simulink model "mdl01_IdealCtrl"  (R2022a)
settings: Solver=FixedStepAuto  StartTime=0.0  StopTime=T1  FixedStep=Ts  RelTol=1e-3
undefined symbols (not defined in the file): a, du, G1, G2, Ts, v0, x0, xt
settings Model: Creator=xiaocy  LastModifiedBy=xiaocy
settings DataIOCC: SaveOutput=off  SignalLogging=off  DSMLogging=off  SaveTime=off  ReturnWorkspaceOutputs=off

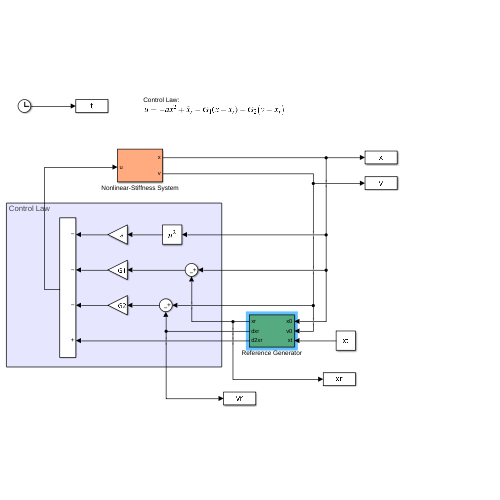
[thumbnail: Simulink's stored preview of the top-level diagram]
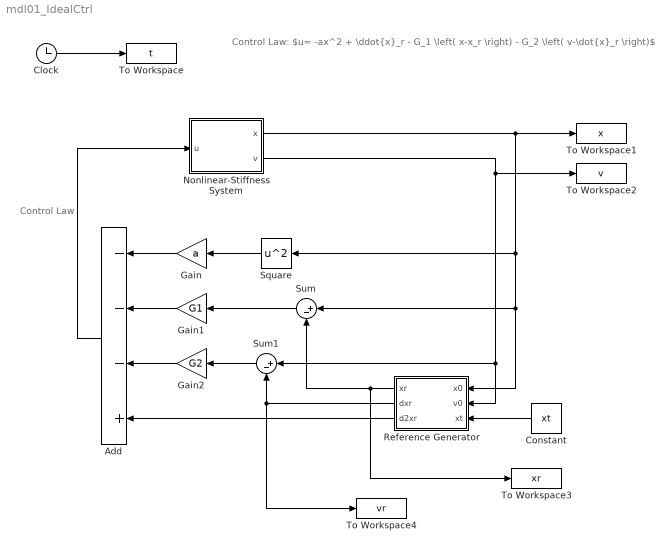
== system mdl01_IdealCtrl ==
  note: Control Law
  note: Control Law:
      | $u= -ax^2 + \ddot{x}_r - G_1 \left( x-x_r \right) - G_2 \left( v-\dot{x}_r \right)$
  Add : Sum  Inputs=---+
  Clock : Clock
  Constant : Constant  Value=xt
  Gain : Gain  Gain=a
  Gain1 : Gain  Gain=G1
  Gain2 : Gain  Gain=G2
  Nonlinear-Stiffness System : Subsystem
  Reference Generator : Subsystem
  Square : Math  Operator=square
  Sum : Sum  Inputs=|+-
  Sum1 : Sum  Inputs=|+-
  To Workspace : ToWorkspace  VariableName=t  SampleTime=Ts
  To Workspace1 : ToWorkspace  VariableName=x  SampleTime=Ts
  To Workspace2 : ToWorkspace  VariableName=v  SampleTime=Ts
  To Workspace3 : ToWorkspace  VariableName=xr  SampleTime=Ts
  To Workspace4 : ToWorkspace  VariableName=vr  SampleTime=Ts
  wires:
  Clock/1 -> To Workspace/1
  Nonlinear-Stiffness System/1(x) -> Sum/1, Reference Generator/1(x0), Square/1, To Workspace1/1
  Nonlinear-Stiffness System/2(v) -> To Workspace2/1, Sum1/1, Reference Generator/2(v0)
  Reference Generator/1(xr) -> To Workspace3/1, Sum/2
  Sum/1 -> Gain1/1
  Sum1/1 -> Gain2/1
  Reference Generator/2(dxr) -> To Workspace4/1, Sum1/2
  Square/1 -> Gain/1
  Gain/1 -> Add/1
  Gain1/1 -> Add/2
  Gain2/1 -> Add/3
  Reference Generator/3(d2xr) -> Add/4
  Add/1 -> Nonlinear-Stiffness System/1(u)
  Constant/1 -> Reference Generator/3(xt)

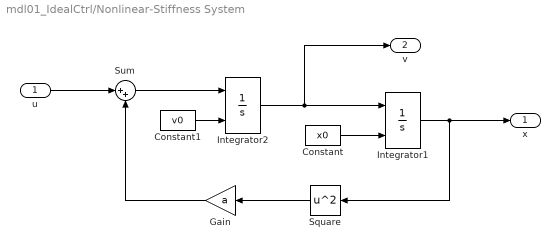
== system mdl01_IdealCtrl/Nonlinear-Stiffness System ==
  u : Inport
  Constant : Constant  Value=x0
  Constant1 : Constant  Value=v0
  Gain : Gain  Gain=a
  Integrator1 : Integrator  InitialConditionSource=external
  Integrator2 : Integrator  InitialConditionSource=external
  Square : Math  Operator=square
  Sum : Sum  Inputs=|++
  x : Outport
  v : Outport  Port=2
  wires:
  Gain/1 -> Sum/2
  Square/1 -> Gain/1
  Sum/1 -> Integrator2/1
  Integrator2/1 -> v/1, Integrator1/1
  u/1 -> Sum/1
  Integrator1/1 -> Square/1, x/1
  Constant/1 -> Integrator1/2
  Constant1/1 -> Integrator2/2

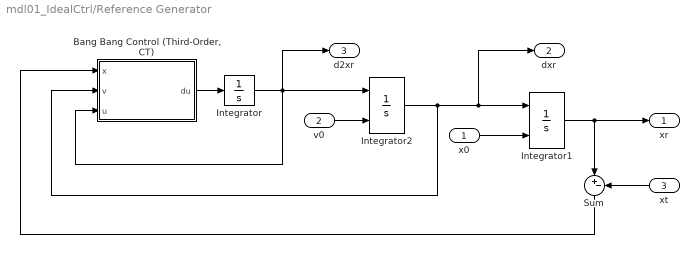
== system mdl01_IdealCtrl/Reference Generator ==
  x0 : Inport
  v0 : Inport  Port=2
  xt : Inport  Port=3
  "Bang Bang Control (Third-Order, CT)" : Subsystem  mask(Bang Bang Control){r=du}
      mask prompts: r "Actuation slope"
      mask help: Calculate command for the third-order system (series of intergrators).
      mask Display: disp('Bang-Bang\n\n(3rd, CT)')
  Integrator : Integrator
  Integrator1 : Integrator  InitialConditionSource=external
  Integrator2 : Integrator  InitialConditionSource=external
  Sum : Sum  Inputs=|+-
  xr : Outport
  dxr : Outport  Port=2
  d2xr : Outport  Port=3
  wires:
  v0/1 -> Integrator2/2
  x0/1 -> Integrator1/2
  Integrator1/1 -> xr/1, Sum/1
  Integrator2/1 -> "Bang Bang Control (Third-Order, CT)"/2(v), Integrator1/1, dxr/1
  Integrator/1 -> Integrator2/1, d2xr/1, "Bang Bang Control (Third-Order, CT)"/3(u)
  "Bang Bang Control (Third-Order, CT)"/1(du) -> Integrator/1
  xt/1 -> Sum/2
  Sum/1 -> "Bang Bang Control (Third-Order, CT)"/1(x)

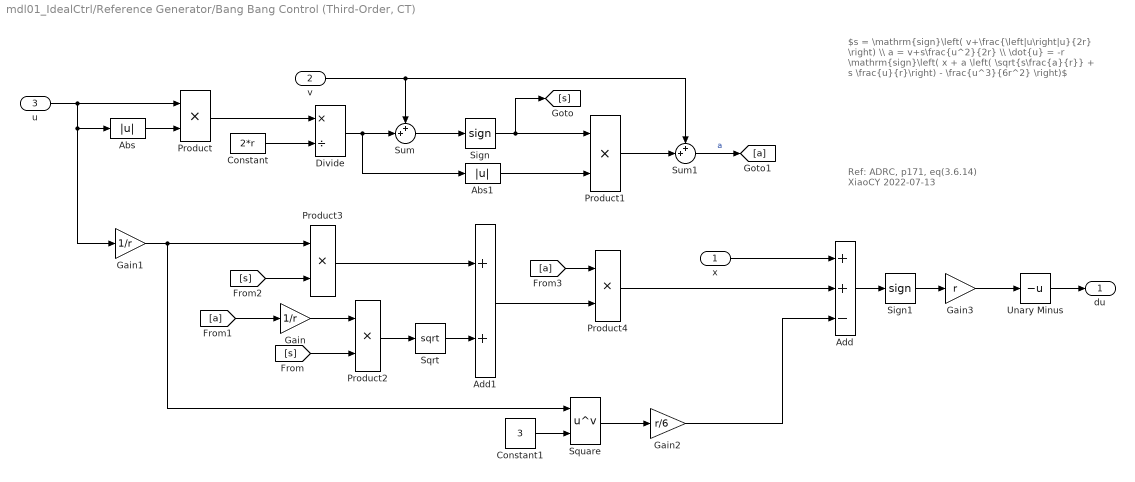
== system mdl01_IdealCtrl/Reference Generator/Bang Bang Control (Third-Order, CT) ==
  note: Ref: ADRC, p171, eq(3.6.14)
      | XiaoCY 2022-07-13
  note: $s = \mathrm{sign}\left( v+\frac{\left|u\right|u}{2r} \right) \\ a = v+s\frac{u^2}{2r} \\ \dot{u} = -r \mathrm{sign}\left( x + a \left( \sqrt{s\frac{a}{r}} + s \frac{u}{r}\right) - \frac{u^3}{6r^2} \right)$
  x : Inport
  v : Inport  Port=2
  u : Inport  Port=3
  Abs : Abs  SaturateOnIntegerOverflow=off
  Abs1 : Abs  SaturateOnIntegerOverflow=off
  Add : Sum  Inputs=++-
  Add1 : Sum
  Constant : Constant  Value=2*r
  Constant1 : Constant  Value=3
  Divide : Product  Inputs=*/
  Gain : Gain  Gain=1/r
  Gain1 : Gain  Gain=1/r
  Gain2 : Gain  Gain=r/6
  Gain3 : Gain  Gain=r
  Product{,1..4} (5 alike) : Product
  Sign : Signum
  Sign1 : Signum
  Sqrt : Sqrt
  Square : Math  Operator=pow
  Sum : Sum  Inputs=++|
  Sum1 : Sum  Inputs=++|
  Unary Minus : UnaryMinus
  du : Outport
  wires:
  u/1 -> Gain1/1, Abs/1, Product/1
  Abs/1 -> Product/2
  Product/1 -> Divide/1
  Constant/1 -> Divide/2
  Divide/1 -> Abs1/1, Sum/2
  Sign/1 -> [s], Product1/1
  Sum/1 -> Sign/1
  v/1 -> Sum1/1, Sum/1
  Abs1/1 -> Product1/2
  Product1/1 -> Sum1/2
  x/1 -> Add/1
  Sum1/1 -> [a]  "a"
  [a] -> Gain/1
  Gain/1 -> Product2/1
  [s] -> Product2/2
  Product2/1 -> Sqrt/1
  Sqrt/1 -> Add1/2
  [s] -> Product3/2
  Gain1/1 -> Square/1, Product3/1
  Product3/1 -> Add1/1
  Add1/1 -> Product4/2
  [a] -> Product4/1
  Product4/1 -> Add/2
  Constant1/1 -> Square/2
  Square/1 -> Gain2/1
  Gain2/1 -> Add/3
  Add/1 -> Sign1/1
  Sign1/1 -> Gain3/1
  Gain3/1 -> Unary Minus/1
  Unary Minus/1 -> du/1
